simulink model "LgrstOpenRStateCtrl"  (R2018b)
settings: Solver=FixedStepDiscrete  StartTime=0.0  StopTime=10.0  FixedStep=0.01  RelTol=1e-3
libraries: StateCtrlLib x1
settings Model: Creator=sn2xws  LastModifiedBy=sn2xws
settings DataIOCC: SaveFormat=StructureWithTime
settings OptimizationCC: DefaultParameterBehavior=Inlined  EnhancedBackFolding=on  PassReuseOutputArgsAs=Individual arguments  ZeroExternalMemoryAtStartup=off  ZeroInternalMemoryAtStartup=off  OptimizeBlockOrder=speed  DifferentSizesBufferReuse=on  OptimizationCustomize=off
settings DebuggingCC: ParameterTunabilityLossMsg=error
settings ModelReferenceCC: ModelReferenceNumInstancesAllowed=Single
settings SFSimCC: MATLABDynamicMemAlloc=off
settings RTWCC: SystemTargetFile=autosar.tlc  GenCodeOnly=on  TemplateMakefile=ert_default_tmf  Description=AUTOSAR  GenerateReport=on  IncludeHyperlinkInReport=on  LaunchReport=on  GenerateTraceInfo=on  GenerateTraceReport=on  GenerateTraceReportSl=on  GenerateTraceReportSf=on  GenerateTraceReportEml=on
settings CodeAppCC: ForceParamTrailComments=on  IgnoreCustomStorageClasses=off  OperatorAnnotations=on  SimulinkDataObjDesc=on  SFDataObjDesc=on  InsertBlockDesc=on
settings STFCustomTargetCC: TargetLangStandard=C99 (ISO)  MultiwordLength=256  ParMdlRefBuildCompliant=on  CompOptLevelCompliant=on  IncludeMdlTerminateFcn=off  CombineOutputUpdateFcns=on  SuppressErrorStatus=on  ERTCustomFileBanners=on  SupportNonFinite=off  SupportComplex=off  SupportContinuousTime=off  SupportNonInlinedSFcns=off  RemoveResetFunc=on  MATLABClassNameForMDSCustomization=Simulink.SoftwareTarget.ERTCustomization  AutosarCompliant=on  UseToolchainInfoCompliant=on  LookupTableObjectStructAxisOrder=2,1,3,4,...  LUTObjectStructOrderEvenSpacing=Size,Table,Breakpoints  SystemTargetFile=autosar.tlc
settings ERTTargetCC: TargetLangStandard=C99 (ISO)  ConcurrentExecutionCompliant=off  IncludeMdlTerminateFcn=off  SuppressErrorStatus=on  SupportNonFinite=off  SupportComplex=off  ModelStepFunctionPrototypeControlCompliant=off  CPPClassGenCompliant=off  AutosarCompliant=on  LookupTableObjectStructAxisOrder=2,1,3,4,...  LUTObjectStructOrderEvenSpacing=Size,Table,Breakpoints  InlinedParameterPlacement=NonHierarchical  ERTCustomFileTemplate=example_file_process.tlc

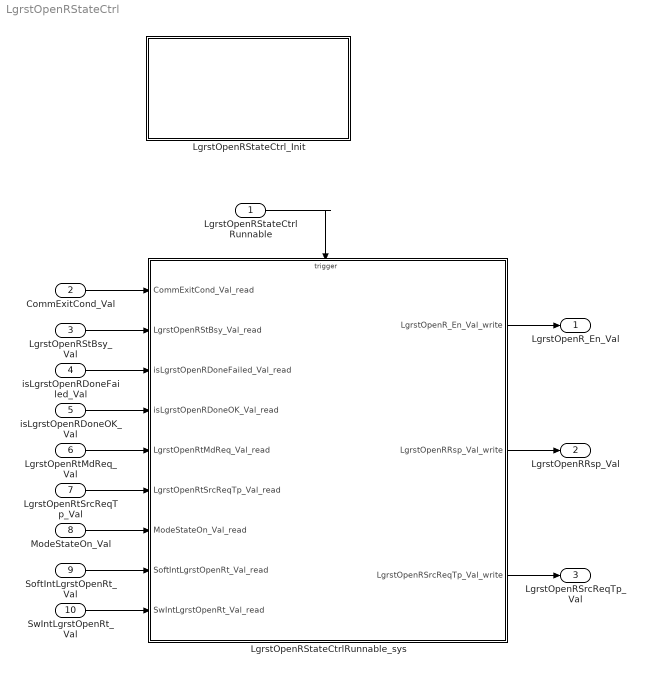
== system LgrstOpenRStateCtrl ==
  LgrstOpenRStateCtrlRunnable : Inport  SampleTime=0.01  OutputFunctionCall=on
  CommExitCond_Val : Inport  Port=2  OutDataTypeStr=boolean  PortDimensions=1
  LgrstOpenRStBsy_Val : Inport  Port=3  OutDataTypeStr=boolean  PortDimensions=1
  isLgrstOpenRDoneFailed_Val : Inport  Port=4  OutDataTypeStr=boolean  PortDimensions=1
  isLgrstOpenRDoneOK_Val : Inport  Port=5  OutDataTypeStr=boolean  PortDimensions=1
  LgrstOpenRtMdReq_Val : Inport  Port=6  OutDataTypeStr=boolean  PortDimensions=1
  LgrstOpenRtSrcReqTp_Val : Inport  Port=7  OutDataTypeStr=Enum: SrcReqTp1  PortDimensions=1
  ModeStateOn_Val : Inport  Port=8  OutDataTypeStr=boolean  PortDimensions=1
  SoftIntLgrstOpenRt_Val : Inport  Port=9  OutDataTypeStr=IntEnable  PortDimensions=1
  SwIntLgrstOpenRt_Val : Inport  Port=10  OutDataTypeStr=IntEnable  PortDimensions=1
  LgrstOpenRStateCtrlRunnable_sys : Subsystem
  LgrstOpenRStateCtrl_Init : Subsystem
  LgrstOpenR_En_Val : Outport  OutDataTypeStr=boolean  PortDimensions=1
  LgrstOpenRRsp_Val : Outport  Port=2  OutDataTypeStr=Enum: MdRspLocal1  PortDimensions=1
  LgrstOpenRSrcReqTp_Val : Outport  Port=3  OutDataTypeStr=Enum: SrcReqTp1  PortDimensions=1
  wires:
  CommExitCond_Val/1 -> LgrstOpenRStateCtrlRunnable_sys/1(CommExitCond_Val_read)
  LgrstOpenRStBsy_Val/1 -> LgrstOpenRStateCtrlRunnable_sys/2(LgrstOpenRStBsy_Val_read)
  isLgrstOpenRDoneFailed_Val/1 -> LgrstOpenRStateCtrlRunnable_sys/3(isLgrstOpenRDoneFailed_Val_read)
  isLgrstOpenRDoneOK_Val/1 -> LgrstOpenRStateCtrlRunnable_sys/4(isLgrstOpenRDoneOK_Val_read)
  LgrstOpenRtMdReq_Val/1 -> LgrstOpenRStateCtrlRunnable_sys/5(LgrstOpenRtMdReq_Val_read)
  LgrstOpenRtSrcReqTp_Val/1 -> LgrstOpenRStateCtrlRunnable_sys/6(LgrstOpenRtSrcReqTp_Val_read)
  ModeStateOn_Val/1 -> LgrstOpenRStateCtrlRunnable_sys/7(ModeStateOn_Val_read)
  SoftIntLgrstOpenRt_Val/1 -> LgrstOpenRStateCtrlRunnable_sys/8(SoftIntLgrstOpenRt_Val_read)
  SwIntLgrstOpenRt_Val/1 -> LgrstOpenRStateCtrlRunnable_sys/9(SwIntLgrstOpenRt_Val_read)
  LgrstOpenRStateCtrlRunnable_sys/1(LgrstOpenR_En_Val_write) -> LgrstOpenR_En_Val/1
  LgrstOpenRStateCtrlRunnable_sys/2(LgrstOpenRRsp_Val_write) -> LgrstOpenRRsp_Val/1
  LgrstOpenRStateCtrlRunnable_sys/3(LgrstOpenRSrcReqTp_Val_write) -> LgrstOpenRSrcReqTp_Val/1
  LgrstOpenRStateCtrlRunnable/1 -> LgrstOpenRStateCtrlRunnable_sys/Trigger

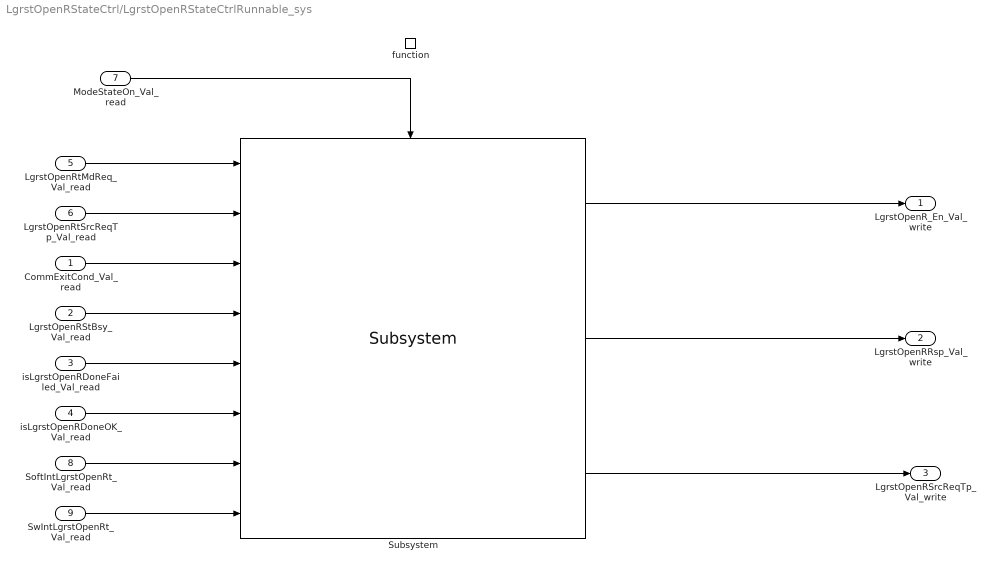
== system LgrstOpenRStateCtrl/LgrstOpenRStateCtrlRunnable_sys ==
  CommExitCond_Val_read : Inport
  LgrstOpenRStBsy_Val_read : Inport  Port=2
  isLgrstOpenRDoneFailed_Val_read : Inport  Port=3
  isLgrstOpenRDoneOK_Val_read : Inport  Port=4
  LgrstOpenRtMdReq_Val_read : Inport  Port=5
  LgrstOpenRtSrcReqTp_Val_read : Inport  Port=6
  ModeStateOn_Val_read : Inport  Port=7
  SoftIntLgrstOpenRt_Val_read : Inport  Port=8
  SwIntLgrstOpenRt_Val_read : Inport  Port=9
  function : TriggerPort  TriggerType=function-call  VariantControl=(inherit)  SampleTimeType=periodic  SampleTime=-1
  Subsystem : StateCtrlLib/Subsystem  SystemSampleTime=-1
  LgrstOpenR_En_Val_write : Outport
      settings: EnsureOutportIsVirtual=on
  LgrstOpenRRsp_Val_write : Outport  Port=2
      settings: EnsureOutportIsVirtual=on
  LgrstOpenRSrcReqTp_Val_write : Outport  Port=3
      settings: EnsureOutportIsVirtual=on
  wires:
  Subsystem/1 -> LgrstOpenR_En_Val_write/1
  Subsystem/2 -> LgrstOpenRRsp_Val_write/1
  Subsystem/3 -> LgrstOpenRSrcReqTp_Val_write/1
  ModeStateOn_Val_read/1 -> Subsystem/Enable
  LgrstOpenRtMdReq_Val_read/1 -> Subsystem/1
  CommExitCond_Val_read/1 -> Subsystem/3
  LgrstOpenRStBsy_Val_read/1 -> Subsystem/4
  LgrstOpenRtSrcReqTp_Val_read/1 -> Subsystem/2
  isLgrstOpenRDoneFailed_Val_read/1 -> Subsystem/5
  SoftIntLgrstOpenRt_Val_read/1 -> Subsystem/7
  isLgrstOpenRDoneOK_Val_read/1 -> Subsystem/6
  SwIntLgrstOpenRt_Val_read/1 -> Subsystem/8

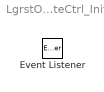
== system LgrstOpenRStateCtrl/LgrstOpenRStateCtrl_Init ==
  Event Listener : EventListener  EventName=reset
